simulink model "FuzzySugenoPID_SingleTank"  (Simulink 10.2)
settings: Solver=ode5  StartTime=0.0  StopTime=600  FixedStep=0.1  MaxStep=0.1  RelTol=1e-3
PreLoadFcn:
  | FuzzyK=readfis('FuzzySugenoPID_SingleTank.fis');
StartFcn:
  | FuzzyK=readfis('FuzzySugenoPID_SingleTank.fis');
undefined symbols (not defined in the file): sigbuilder_block
libraries: fuzblock x1
Description:
  | The model describes dynamic properties of tank level system. The differential equation is:
  |                                            d/dt{Ah(t))=ku(t)-a*sqrt(2*g*h(t))
settings Model: Creator=Huynh Thai Hoang  LastModifiedBy=TBL  ExtModeTrigMode=oneshot  ExtModeArmWhenConnect=off
settings SolverCC: InitialStep=0.1
settings DataIOCC: SaveOutput=off  SaveTime=off  SignalLoggingName=sigsOut
settings OptimizationCC: BooleanDataType=off  ExpressionDepthLimit=2147483647
settings DebuggingCC: SaveWithParameterizedLinksMsg=none  SignalResolutionControl=TryResolveAllWithWarning  MultiTaskDSMMsg=warning  MultiTaskCondExecSysMsg=none  StateNameClashWarn=warning
settings HardwareCC: TargetUnknown=on

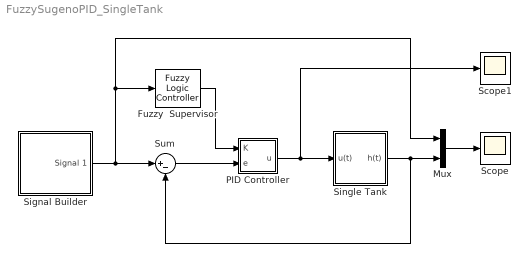
== system FuzzySugenoPID_SingleTank ==
  Fuzzy  Supervisor : fuzblock/Fuzzy Logic  Controller  FIS=FuzzyK  OutputSampleNumber=101  DataType=double  FuzzifiedInputs=off  RuleFiringStrengths=off  RuleOutputs=off  AggregatedOutputs=off  SimulateUsing=Interpreted execution  OutOfRangeInputValueMessage=warning  NoRuleFiredMessage=warning  EmptyOutputFuzzySetMessage=warning
  Mux : Mux  Inputs=2
  PID Controller : Subsystem  AncestorBlock=simulink_extras/Additional Linear/PID Controller  mask(PID Controller){}
      mask help:
      | Enter expressions for proportional, integral, and derivative terms.
      | P+I/s+Ds
      mask Help: This block implements a PID controller where parameters are entered for the Proportional, Integral and Derivative terms. Unmask this block to see how it works. The derivative term is implemented using a true derivative block.
  Scope : Scope
  Scope1 : Scope
  Signal Builder : Subsystem  Tag=STV Subsys  LoadFcn=sigbuilder_block('load');  StartFcn=sigbuilder_block('start');  StopFcn=sigbuilder_block('stop');  ClipboardFcn=sigbuilder_block('clipboard');  mask(Sigbuilder block){tuvar=[0:10]}
      mask help: Create and generate interchangeable groups of signals whose waveforms are piecewise linear.
      mask init:
      | if ~strcmp(get_param(bdroot(gcbh),'SimulationStatus'),'stopped') tuvar = sigbuilder_block('maskInit'); end
      settings: CopyFcn=sigbuilder_block('copy');  DeleteFcn=sigbuilder_block('delete');  ModelCloseFcn=sigbuilder_block('modelClose');  PreSaveFcn=sigbuilder_block('preSave');  PauseFcn=sigbuilder_block('pause')  ContinueFcn=sigbuilder_block('continue')  NameChangeFcn=sigbuilder_block('namechange');  OpenFcn=sigbuilder_block('open',[112.5 99 550.5 394.5 ]);  CloseFcn=sigbuilder_block('close');
      mask Display: plot(0, 0, 100, 100,[2, 2, 32, 32, 2], [68, 8, 8, 68, 68],[32, 2], [38, 38], [32, 19, 2],[53, 60, 44], [32, 17, 17, 2],[16, 16, 31, 31]);txt = getActiveGroup(gcbh);text(2, 100, txt,'verticalAlignment', 'top');
  Single Tank : Subsystem  mask{A_min=50, A_max=200, a_out=1, h_max=50, Q_max=300, U_max=12, C=0.6}
      mask prompts: A_min "Minimum cross area (cm2)"; A_max "Maximum cross area (cm2)"; a_out "Outlet area (cm2)"; h_max "Tank height (cm)"; Q_max "Maximum pump flow (cm3/sec)"; U_max "Maximum control voltage (V)"; C "Discharge constant"
      mask init:
      | g=981;
      | k=Q_max/U_max;
      mask Display:
      | plot([0.1 0.3 0.9],[0.9 0.1 0.1]);
      | plot([0.9 0.7 0.9],[0.9 0.2 0.2]);
  Sum : Sum  Inputs=|+-  SaturateOnIntegerOverflow=on
  wires:
  Signal Builder/1(Signal 1) -> Sum/1, Mux/1, Fuzzy  Supervisor/1
  Sum/1 -> PID Controller/2(e)
  PID Controller/1(u) -> Single Tank/1(u(t)), Scope1/1
  Single Tank/1(h(t)) -> Sum/2, Mux/2
  Fuzzy  Supervisor/1 -> PID Controller/1(K)
  Mux/1 -> Scope/1

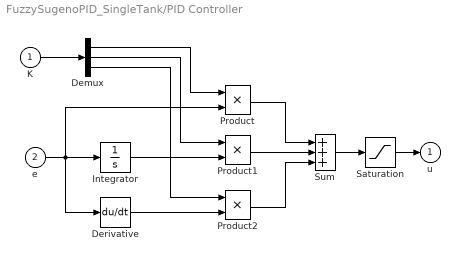
== system FuzzySugenoPID_SingleTank/PID Controller ==
  K : Inport
  e : Inport  Port=2
  Demux : Demux  Outputs=3
      settings: DisplayOption=none
  Derivative : Derivative
  Integrator : Integrator
  Product : Product  SaturateOnIntegerOverflow=on  OutDataTypeStr=Inherit: Same as first input
  Product1 : Product  SaturateOnIntegerOverflow=on  OutDataTypeStr=Inherit: Same as first input
  Product2 : Product  SaturateOnIntegerOverflow=on  OutDataTypeStr=Inherit: Same as first input
  Saturation : Saturate  UpperLimit=12  LowerLimit=0
  Sum : Sum  Inputs=+++  InputSameDT=on  SaturateOnIntegerOverflow=on  OutDataTypeStr=Inherit: Same as first input
  u : Outport  InitialOutput=0
  wires:
  Product/1 -> Sum/1
  e/1 -> Product/2, Integrator/1, Derivative/1
  Sum/1 -> Saturation/1
  K/1 -> Demux/1
  Demux/1 -> Product/1
  Product1/1 -> Sum/2
  Integrator/1 -> Product1/2
  Demux/2 -> Product1/1
  Derivative/1 -> Product2/2
  Product2/1 -> Sum/3
  Demux/3 -> Product2/1
  Saturation/1 -> u/1

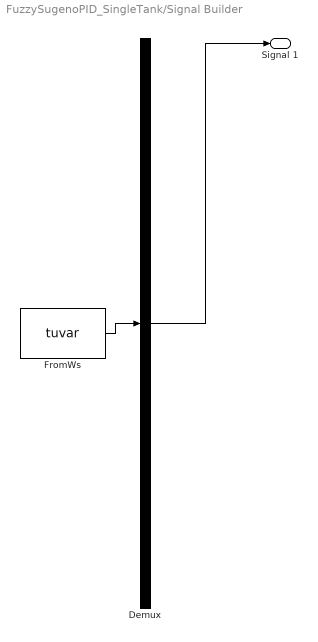
== system FuzzySugenoPID_SingleTank/Signal Builder ==
  Demux : Demux  Tag=STV Demux  Outputs=1
      settings: DisplayOption=none
  FromWs : FromWorkspace  Tag=STV FromWs  VariableName=tuvar  SigBuilderData=DataTag0  VnvData=DataTag1
      SigBuilderData=|
      | common.afterFinalStr = 'Extrapolate'
      | common.sampleTime = 0
      | dataSet.timeRange = [0 600]
      | dataSet.name = 'Group 1'
      | sbobj.Groups.Name = 'Group 1'
      | sbobj.Groups.Signals.Name = 'Signal 1'
      | sbobj.Groups.Signals.XData = [0 101 101 202 202 327 327 458 458 600]
      | sbobj.Groups.Signals.YData = [9.8 9.8 17.6 17.6 5.2 5.2 25.8 25.8 20 20]
      | sbobj.Groups.TimeRange = [0 600]
  Signal 1 : Outport  Tag=STV Outport
  wires:
  Demux/1 -> Signal 1/1
  FromWs/1 -> Demux/1

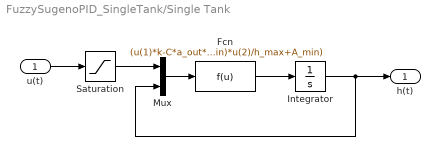
== system FuzzySugenoPID_SingleTank/Single Tank ==
  u(t) : Inport
  Fcn : Fcn  Expr=(u(1)*k-C*a_out*sqrt(2*g*u(2)))/((A_max-A_min)*u(2)/h_max+A_min)
  Integrator : Integrator  LimitOutput=on  UpperSaturationLimit=h_max  LowerSaturationLimit=0
  Mux : Mux  Inputs=2
  Saturation : Saturate  UpperLimit=12  LowerLimit=0
  h(t) : Outport
  wires:
  u(t)/1 -> Saturation/1
  Mux/1 -> Fcn/1
  Fcn/1 -> Integrator/1
  Integrator/1 -> h(t)/1, Mux/2
  Saturation/1 -> Mux/1
